simulink model "Simulacion_stepper"  (R2025b)
settings: Solver=ode4  StartTime=0.0  StopTime=Time_simulation  FixedStep=1/frecuency_simulation  RelTol=1e-3
InitFcn:
  | %%InitFcn();
StopFcn:
  | %%FinishFcn
model workspace (MAT data in the model file):
  Ts_stepper = 0.001
values from neighbouring files (symbols this model uses):
  B = motor_params.B_internal    [bode.m]    (also in current_observer.m = 0.0005; discretizacion.m = [ 1/L, 0; ekf_4_estados.m = params.B; obs_ctrl_back_emf_ext.m = [1/L 0)
  frecuency_simulation = 10e3    (= 10000)    [InitFcn.m]
  J = motor_params.J_internal    [bode.m]    (also in current_observer.m = 0.008; ekf_4_estados.m = params.J; obs_ctrl_back_emf_ext.m = 0.008; obs_y_contrl_back_emd.m = 0.008)
  Ke = 0.0055    [current_observer.m]    (also in ekf_4_estados.m = params.Ke; observer.m = Pvec(3); salient_motor.m = 0.0066)
  Ki_d = PI_dq_params.Ki_d_salient    [bode.m]
  Ki_q = PI_dq_params.Ki_q_salient    [bode.m]
  Ki_w = (wn_w^2)*J_var/Kt    [Barrido_B.m]    (also in Barrido_J.m; bode.m = PI_MTPA_params.Ki_w)
  Kp_d = PI_dq_params.Kp_d_salient    [bode.m]
  Kp_q = PI_dq_params.Kp_q_salient    [bode.m]
  Kp_w = (2*shi_w*wn_w*J_var)/Kt    [Barrido_B.m]    (also in Barrido_J.m; bode.m = PI_MTPA_params.Kp_w)
  Kt = Nr*Ke    (= 0.275)    [current_observer.m]    (also in ekf_4_estados.m = params.Kt; frecuencia_max.m = 0.33; observer.m = Pvec(4); salient_motor.m = 0.33)
  L = place(A', C', 10*eig(A)).'    [current_observer.m]    (also in desfase.m = lags(k); discretizacion.m = 0.01; frecuencia_max.m = 0.006; obs_ctrl_back_emf_ext.m = 0.006)
  P = motor_params.P    [bode.m]    (also in ekf_4_estados.m = P_pred; frecuencia_max.m = 50; salient_motor.m = 50)
  R = motor_params.R    [bode.m]    (also in current_observer.m = 3.4; discretizacion.m = 3.4; ekf_4_estados.m = params.R; frecuencia_max.m = 3.4)
  sample_time = 1/frecuency_simulation    (= 0.0001)    [InitFcn.m]
  Ts_current = 1/f_current    (= 0.0001)    [InitFcn.m]
  Ts_Wm = Ts_current*10    (= 0.001)    [InitFcn.m]
  Vdc = 24    [InitFcn.m]    (also in frecuencia_max.m = 12)
undefined symbols (not defined in the file or in its folder): DiscIntNeverNeededParam, EKF_params, motor_params, RI_base
libraries: simulink x8, mcbeeMathTransformLib x3, spspowerguiLib x1
(part 1 of 5)
settings Model: DataTypeOverride=Off  SimulationMode=accelerator  Creator=PC  LastModifiedBy=damia
settings DataIOCC: Decimation=20
settings OptimizationCC: OptimizeBlockIOStorage=off  SimCompilerOptimization=on  OptimizeDataStoreBuffers=off  BusAssignmentInplaceUpdate=off  UseRowMajorAlgorithm=on
settings DebuggingCC: SFUnexpectedBacktrackingDiag=warning  SFNoUnconditionalDefaultTransitionDiag=warning  UnderSpecifiedDimensionMsg=warning
settings RTWCC: GenerateReport=on  BuildConfiguration=Debug  LaunchReport=on
settings CodeAppCC: ForceParamTrailComments=on  MATLABSourceComments=on  EnableCustomComments=on
settings GRTTargetCC: MultiInstanceErrorCode=Warning  CombineSignalStateStructs=on  SupportVariableSizeSignals=on
settings SimscapeCC: ExplicitSolverDiagnosticOptions=none

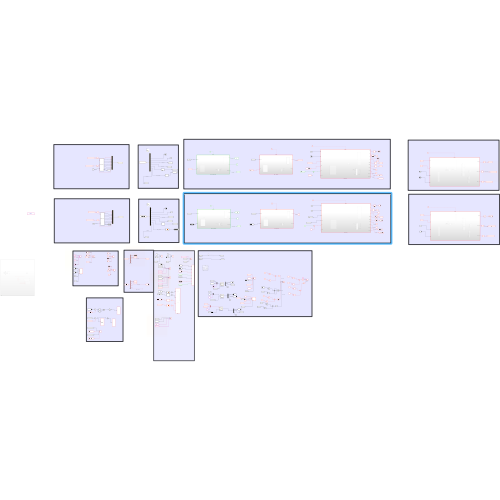
[thumbnail: Simulink's stored preview of the top-level diagram]
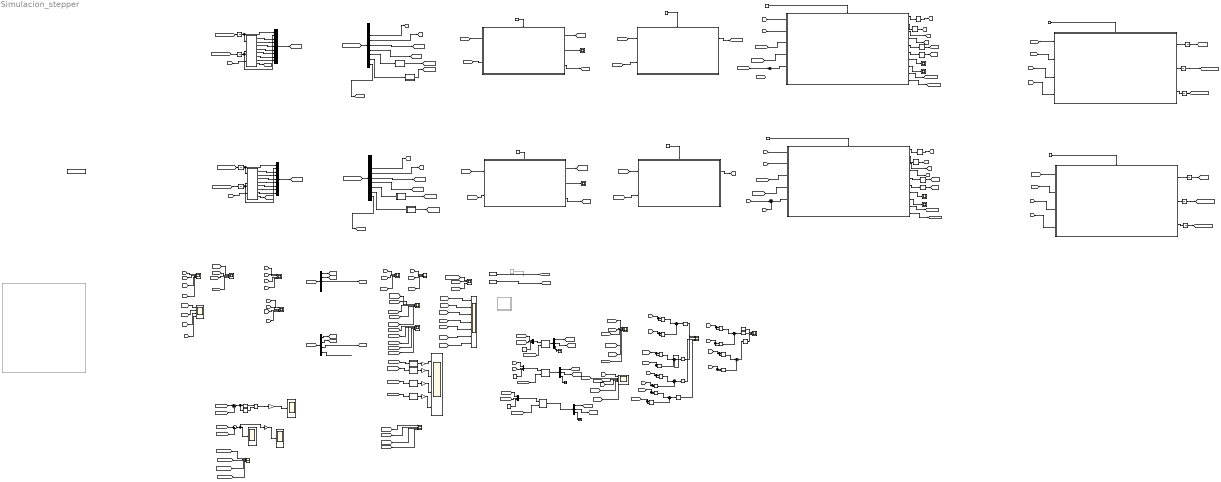
== system Simulacion_stepper ==
  note: Vab
      | Iab,
      | Te(N*m),
      | We(rad/s),
      | Theta_e(rad)
  note: Vab
      | Iab,
      | Te(N*m),
      | We(rad/s),
      | Theta_e(rad)
  Atan1 : Trigonometry  Operator=atan2
  Clarke to Park Angle Transform : mcbeeMathTransformLib/Clarke to Park Angle Transform  AxisAlignment=D-axis  UseWithEmbedded=off  PhaseInput=Two inputs  ThetaInput=Sine and Cosine electrical position  AngleInput=Per-unit  N_points=1024
      settings: LibrarySourceBlock=|
      | ee_sl_lib/Mathematical
      | Transforms/Clarke to Park
      | Angle Transform
  Clarke to Park Angle Transform1 : mcbeeMathTransformLib/Clarke to Park Angle Transform  AxisAlignment=D-axis  UseWithEmbedded=off  PhaseInput=Two inputs  ThetaInput=Sine and Cosine electrical position  AngleInput=Per-unit  N_points=1024
      settings: LibrarySourceBlock=|
      | ee_sl_lib/Mathematical
      | Transforms/Clarke to Park
      | Angle Transform
  Constant1 : Constant  Value=Vdc
  Constant11 : Constant  Value=0  OutDataTypeStr=double
  Constant2 : Constant  Value=0  OutDataTypeStr=double
  Constant6 : Constant  Value=0  OutDataTypeStr=double
  Cos1 : Trigonometry  Operator=cos
  Demux : Demux  Outputs=9
  Demux1 : Demux  Outputs=3
  Demux2 : Demux  Outputs=3
  Demux3 : Demux  Outputs=9
  Demux5 : Demux  Outputs=3
  Function-Call Generator : FunctionCallGenerator  SampleTime=EKF_params.Ts
  Function-Call Generator1 : FunctionCallGenerator  SampleTime=EKF_params.Ts
  Function-Call Generator10 : FunctionCallGenerator  Commented=on  SampleTime=1/1000
  Function-Call Generator13 : FunctionCallGenerator  SampleTime=RI_base.Ts
  Function-Call Generator2 : FunctionCallGenerator  SampleTime=RI_base.Ts
  Function-Call Generator3 : FunctionCallGenerator  SampleTime=Ts_current
  Function-Call Generator4 : FunctionCallGenerator  SampleTime=Ts_current
  Function-Call Generator5 : FunctionCallGenerator  SampleTime=Ts_Wm
  Function-Call Generator6 : FunctionCallGenerator  SampleTime=Ts_Wm
  Gain{1,25..26,28,30} (5 alike) : Gain  Gain=180/pi
  Gain2 : Gain  Gain=motor_params.P
  Iab : Scope  NumInputPorts=4
      settings: ActiveDisplayYMinimum=-2.7580893331915077  ActiveDisplayYMaximum=5.9277803516478356  DataLoggingVariableName=ScopeData8
  Id : Scope  NumInputPorts=6
      settings: ActiveDisplayYMinimum=-0.42609115554446897  ActiveDisplayYMaximum=0.9985187345386608  DataLoggingVariableName=ScopeData2
  Idq : Scope  NumInputPorts=4
      settings: ActiveDisplayYMinimum=-1  ActiveDisplayYMaximum=1  DataLoggingVariableName=ScopeData6
  Imag : Scope  NumInputPorts=4
      settings: ActiveDisplayYMinimum=-0.27016077029893221  ActiveDisplayYMaximum=2.4314469326903905  DataLoggingVariableName=ScopeData2
  Iq : Scope  NumInputPorts=6
      settings: ActiveDisplayYMinimum=-0.66469283994282913  ActiveDisplayYMaximum=2.8527838782953632  DataLoggingVariableName=Iq
  Level-2 MATLAB S-Function : M-S-Function  FunctionName=PMSM_salient  Parameters=motor_params
  Level-2 MATLAB S-Function1 : M-S-Function  FunctionName=PMSM_salient  Parameters=motor_params
  MATLAB Function1 : MATLAB Function  TreatAsAtomicUnit=on
  MATLAB Function10 : MATLAB Function  TreatAsAtomicUnit=on
  MATLAB Function12 : MATLAB Function  TreatAsAtomicUnit=on
  MATLAB Function14 : MATLAB Function  TreatAsAtomicUnit=on
  MATLAB Function3 : MATLAB Function  TreatAsAtomicUnit=on
  MATLAB Function4 : MATLAB Function  TreatAsAtomicUnit=on
  MATLAB Function5 : MATLAB Function  TreatAsAtomicUnit=on
  MATLAB Function9 : MATLAB Function  TreatAsAtomicUnit=on
  Motor 1  Speed PR : Subsystem  TreatAsAtomicUnit=on
  Motor 2  Speed PR : Subsystem  TreatAsAtomicUnit=on
  Motor 2 PI Speed MTPA : Subsystem  TreatAsAtomicUnit=on
  Motor 2 PI Speed MTPA2 : Subsystem  TreatAsAtomicUnit=on
  Motor 2 PI dq : Subsystem  TreatAsAtomicUnit=on
  Motor 2 PI dq1 : Subsystem  TreatAsAtomicUnit=on
  Mux1 : Mux  Inputs=9
  Mux2 : Mux  Inputs=3
  Mux3 : Mux  Inputs=3
  Mux4 : Mux  Inputs=9
  Mux5 : Mux  Inputs=3
  Park to Clarke Angle Transform : mcbeeMathTransformLib/Park to Clarke Angle Transform  AxisAlignment=D-axis  UseWithEmbedded=off  PhaseInput=Two inputs  ThetaInput=Sine and Cosine electrical position  AngleInput=Per-unit  N_points=1024
      settings: LibrarySourceBlock=|
      | ee_sl_lib/Mathematical
      | Transforms/Park to Clarke
      | Angle Transform
  Product{,1..7,14..17} (12 alike) : Product
  Rate Transition{1..8} (8 alike) : RateTransition
  Scope{1,3,7..8,10..11,14..15,18} (9 alike) : Scope
      Scope1 settings: ActiveDisplayYMinimum=-1  ActiveDisplayYMaximum=1  DataLoggingVariableName=ScopeData13
      Scope10 settings: ActiveDisplayYMinimum=-28.272805787309412  ActiveDisplayYMaximum=20.9806919386897  DataLoggingVariableName=ScopeData15
      Scope11 settings: ActiveDisplayYMinimum=-12246.521454579266  ActiveDisplayYMaximum=6009.4483803605362  DataLoggingVariableName=ScopeData18
      Scope14 settings: ActiveDisplayYMinimum=-21.63251363440429  ActiveDisplayYMaximum=12.126898976697245
      Scope15 settings: ActiveDisplayYMinimum=-3.7842974391773385  ActiveDisplayYMaximum=5.2532390639650686
      Scope18 settings: ActiveDisplayYMinimum=-1  ActiveDisplayYMaximum=1  DataLoggingVariableName=ScopeData14
      Scope3 settings: ActiveDisplayYMinimum=-25.99232285218147  ActiveDisplayYMaximum=26.712868682551036  DataLoggingVariableName=ScopeData10
      Scope7 settings: ActiveDisplayYMinimum=-28.272805787309412  ActiveDisplayYMaximum=20.9806919386897  DataLoggingVariableName=ScopeData11
      Scope8 settings: ActiveDisplayYMinimum=-25.99232285218147  ActiveDisplayYMaximum=26.712868682551036  DataLoggingVariableName=ScopeData17
  Scope12 : Scope  NumInputPorts=3
      settings: ActiveDisplayYMinimum=-0.46724306234141394  ActiveDisplayYMaximum=0.44219800668257625  DataLoggingVariableName=ScopeData2
  Scope2 : Scope  NumInputPorts=7
      settings: ActiveDisplayYMinimum=-3.4057486074692189  ActiveDisplayYMaximum=17.21642789399754
  Scope4 : Scope  NumInputPorts=4
      settings: ActiveDisplayYMinimum=-0.031489749327242751  ActiveDisplayYMaximum=0.031489751273901176  DataLoggingVariableName=ScopeData12
  Scope5 : Scope  NumInputPorts=5
      settings: ActiveDisplayYMinimum=-0.11835861027046617  ActiveDisplayYMaximum=0.88581558269388327
  Scope6 : Scope  NumInputPorts=3
      settings: ActiveDisplayYMinimum=-2.72699  ActiveDisplayYMaximum=4.80249
  Scope9 : Scope  NumInputPorts=4
      settings: ActiveDisplayYMinimum=-0.078542596521209512  ActiveDisplayYMaximum=0.051240487920084017  DataLoggingVariableName=ScopeData16
  Sin1 : Trigonometry
  Sqrt{,1..5} (6 alike) : Sqrt
  Subsystem1 : Subsystem  Commented=on
  Sum{1..6,13..14} (8 alike) : Sum  Inputs=|++
  Sum7 : Sum  Inputs=|+-
  Sum9 : Sum  Inputs=|+-
  Te : Scope  NumInputPorts=5
      settings: ActiveDisplayYMinimum=-0.031497005621000287  ActiveDisplayYMaximum=0.029140494372188255  DataLoggingVariableName=ScopeData2
  Terminator1 : Terminator
  Terminator2 : Terminator
  Terminator3 : Terminator
  Theta_e : Scope  NumInputPorts=4
      settings: ActiveDisplayYMinimum=-308.70038006354309  ActiveDisplayYMaximum=202.06256848293435
  Triggered Subsystem : Subsystem  Commented=on  TreatAsAtomicUnit=on
  Triggered Subsystem1 : Subsystem  TreatAsAtomicUnit=on  DataTypeOverride=Single
  Triggered Subsystem2 : Subsystem  TreatAsAtomicUnit=on  DataTypeOverride=Single
  Unit Delay{1..10} (10 alike) : UnitDelay  SampleTime=-1  HasFrameUpgradeWarning=on
  Vab : Scope  NumInputPorts=4
      settings: ActiveDisplayYMinimum=-4.125  ActiveDisplayYMaximum=4.125  DataLoggingVariableName=ScopeData7
  Valpha_betha : Scope  NumInputPorts=4
      settings: ActiveDisplayYMinimum=-2.9999999999999991  ActiveDisplayYMaximum=27  DataLoggingVariableName=ScopeData3
  Vdq : Scope  NumInputPorts=4
      settings: ActiveDisplayYMinimum=-12.409092353940933  ActiveDisplayYMaximum=27.623166475378763  DataLoggingVariableName=ScopeData5
  Vmag : Scope  NumInputPorts=3
      settings: ActiveDisplayYMinimum=-2.9178979771997589  ActiveDisplayYMaximum=26.435321997466648  DataLoggingVariableName=ScopeData3
  We : Scope  NumInputPorts=3
      settings: ActiveDisplayYMinimum=72.111947362295382  ActiveDisplayYMaximum=388.0476080584769  DataLoggingVariableName=ScopeData4
  Wm_ref : FromWorkspace  VariableName=Wm_ref  Interpolate=off  OutputAfterFinalValue=Holding final value
  Wm_ref3 : FromWorkspace  VariableName=Tl  Interpolate=off  OutputAfterFinalValue=Holding final value
  ekf_4var1 : Demux
  ekf_4var2 : Demux  Outputs=5
  powergui : spspowerguiLib/powergui  Priority=1  SimulationMode=Discrete  SampleTime=1/frecuency_simulation  frequency=60  Iterations=50  frequencyindice=0  Pbase=100e6  ErrMax=1e-4  UnitsV=kV  UnitsW=MW  buscounter=0  FunctionMessages=off  echomessages=off  EnableUseOfTLC=off  CurrentSourceSwitches=off  DisableSnubberDevices=off  DisableRonSwitches=off  DisableVfSwitches=off  DisplayEquations=off  AutomaticDiscreteSolvers=off  SolverType=Tustin/Backward Euler (TBE)  Interpol=off  ExternalGateDelay=off  methode=off  Ts=100  x0status=blocks  SPID=on  SwTol=0  HookPort=off  NonlinearTolerance=1e-4  nMaxIteration=100  ContinueOnMaxIteration=off  RestoreLinks=warning  ResistiveCurrentMeasurement=off  Frange=[0:2:500]  Ylog=off  Xlog=on  ShowGrid=off  save=off  variable=ZData  structure=0  ZoomFFT=off  StartTime=0.0  cycles=1  DisplayStyle=1  fundamental=60  FreqAxis=off  MaxFrequency=1000  frequencyindicesteady=1  RmsSteady=1  display=off
  tag scope: T_ref=global, T_ref_M1=global, Te_planta_M1=global, Te_planta_M2=global, We_planta_M1=global, We_planta_M2=global, Wm_planta_M1=global, Wm_planta_M2=global, theta_e_planta_M1=global, theta_e_planta_M2=global
  wires:
  [Te_planta_M1] -> Te/1
  [We_planta_M1] -> We/2
  [Vd_M1] -> Vdq/1  "Vd_M1"
  [Iq_M1] -> Idq/2  "Iq_M1"
  [Id_M1] -> Idq/1  "Id_M1"
  [Vq_M1] -> Vdq/2  "Vq_M1"
  [Ia_M1] -> Mux2/1
  [Ib_M1] -> Mux2/2
  Constant11/1 -> Mux2/3
  Mux2/1 -> Clarke to Park Angle Transform1/1
  Clarke to Park Angle Transform1/1 -> Demux2/1
  Demux2/3 -> Terminator1/1
  [Iq_M1] -> Iq/1
  [Iq_ref_M1] -> Iq/2
  [Iq_M1] -> Product/2, Product/1
  [Id_M1] -> Product1/2, Product1/1
  Product/1 -> Sum13/1
  Product1/1 -> Sum13/2
  Sum13/1 -> Sqrt/1
  Sqrt/1 -> Imag/1  "I_sat_obs_M1"
  Product3/1 -> Sum14/2
  Sum14/1 -> Sqrt1/1
  [Vq_M1] -> Product2/2, Product2/1
  [Vd_M1] -> Product3/2, Product3/1
  Sqrt1/1 -> Vmag/2  "V_sat_M1"
  Product2/1 -> Sum14/1
  Function-Call Generator/1 -> Triggered Subsystem1/Trigger
  [Te_planta_M2] -> Te/2
  [theta_m_planta_M1] -> Scope5/1
  [theta_m_ref] -> Scope5/3
  [Ia_M2] -> Scope6/2
  [Ia_M1] -> Scope6/1
  [Ib_M1] -> Scope12/1
  [Ib_M2] -> Scope12/2
  [Valpha_M1] -> Valpha_betha/1  "Valpha_M1"
  [Vbetha_M1] -> Valpha_betha/2  "Vbetha_M1"
  Constant1/1 -> Vmag/1
  [Vb_M1] -> Vab/2  "Vb_M1"
  [Va_M1] -> Vab/1  "Va_M1"
  [Valpha_M2] -> Valpha_betha/3  "Valpha_M2"
  [Vbetha_M2] -> Valpha_betha/4  "Vbetha_M2"
  [Ib_M1] -> Iab/2  "Ib_M1"
  [Ia_M1] -> Iab/1  "Ia_M1"
  [Vd_M2] -> Vdq/3  "Vd_M2"
  [Vq_M2] -> Vdq/4  "Vq_M2"
  [Id_M2] -> Idq/3  "Id_M2"
  [Iq_M2] -> Idq/4  "Iq_M2"
  [Iq_M2] -> Iq/4
  [Iq_ref_M2] -> Iq/5
  Product4/1 -> Sum1/1
  [Id_M2] -> Product5/2, Product5/1
  Sum1/1 -> Sqrt2/1
  [Iq_M2] -> Product4/2, Product4/1
  Product5/1 -> Sum1/2
  Product7/1 -> Sum2/2
  [Vq_M2] -> Product6/2, Product6/1
  Sum2/1 -> Sqrt3/1
  [Vd_M2] -> Product7/2, Product7/1
  Product6/1 -> Sum2/1
  Sqrt3/1 -> Vmag/3  "V_sat_M2"
  MATLAB Function3/1(y) -> [theta_m_planta_M2]
  MATLAB Function4/1(y) -> [theta_e_planta_M2]
  [Wm_ref] -> Scope2/1
  Function-Call Generator4/1 -> Motor 2 PI dq/Trigger
  Function-Call Generator5/1 -> Motor 2 PI Speed MTPA/Trigger
  [Wm_ref] -> Motor 2 PI Speed MTPA/1(Wm_ref)
  Motor 2 PI dq/3(Id) -> [Id_M2]
  Motor 2 PI dq/4(Iq) -> [Iq_M2]
  [We_planta_M2] -> We/3
  [var_stepper_M2] -> Demux/1
  Demux/3 -> [Ia_M2]
  Demux/4 -> [Ib_M2]
  [We_planta_M0] -> We/1
  [Va_M2] -> Vab/4  "Va_M2"
  [Vb_M2] -> Vab/3  "Vb_M2"
  [Ia_M2] -> Iab/3  "Ia_M2"
  [Ib_M2] -> Iab/4  "Ib_M2"
  ekf_4var1/2 -> [Iq_obs_M2]  "Iq_obs_M2"
  [x_ekf_5var_M2] -> ekf_4var1/1
  ekf_4var1/3 -> [Wm_obs_M2]  "Wm_obs_M2"
  ekf_4var1/1 -> [Id_obs_M2]  "Id_obs_M2"
  [Ia_obs_M2] -> Scope6/3
  [Ib_obs_M2] -> Scope12/3
  [Id_M1] -> Id/1
  [Id_M2] -> Id/4
  [Ib_M2] -> Mux5/2
  Mux5/1 -> Clarke to Park Angle Transform/1
  [Ia_M2] -> Mux5/1
  Constant6/1 -> Mux5/3
  Clarke to Park Angle Transform/1 -> Demux1/1
  Demux1/3 -> Terminator2/1
  Demux2/1 -> [Id_real_M1]  "Id_real_M1"
  Demux2/2 -> [Iq_real_M1]  "Iq_real_M1"
  Demux1/1 -> [Id_real_M2]  "Id_real_M2"
  Demux1/2 -> [Iq_real_M2]  "Iq_real_M2"
  [Iq_real_M1] -> Iq/3
  [Iq_real_M2] -> Iq/6
  [Id_real_M2] -> Id/6
  Product15/1 -> Sum5/2
  [Id_real_M1] -> Product15/2, Product15/1
  [Iq_real_M1] -> Product14/2, Product14/1
  Sum5/1 -> Sqrt4/1
  Product14/1 -> Sum5/1
  Sum6/1 -> Sqrt5/1
  [Id_real_M2] -> Product17/2, Product17/1
  [Iq_real_M2] -> Product16/2, Product16/1
  Product17/1 -> Sum6/2
  Product16/1 -> Sum6/1
  Sqrt4/1 -> Imag/2  "I_sat_real_M1"
  Sqrt5/1 -> Imag/4  "I_sat_real_M2"
  Sqrt2/1 -> Imag/3  "I_sat_obs_M2"
  [theta_e_obs_M2] -> MATLAB Function14/1(u)
  [theta_e_obs_M1] -> MATLAB Function12/1(u)
  [theta_e_planta_M2] -> MATLAB Function10/1(u)
  [theta_e_planta_M1] -> MATLAB Function9/1(u)
  MATLAB Function10/1(y) -> Gain26/1
  MATLAB Function14/1(y) -> Gain30/1
  MATLAB Function12/1(y) -> Gain28/1
  MATLAB Function9/1(y) -> Gain25/1
  Gain25/1 -> Theta_e/1
  Gain26/1 -> Theta_e/2
  Gain28/1 -> Theta_e/3
  Gain30/1 -> Theta_e/4
  [theta_e_planta_M2] -> Clarke to Park Angle Transform/2
  [theta_e_planta_M1] -> Clarke to Park Angle Transform1/2
  [Wm_obs_M1] -> Sum7/2
  [Wm_planta_M1] -> Sum7/1
  Sum7/1 -> Gain2/1, Scope15/1
  Level-2 MATLAB S-Function/1 -> Mux4/3
  Level-2 MATLAB S-Function/2 -> Mux4/4
  Mux4/1 -> [var_stepper_M2]
  Level-2 MATLAB S-Function/3 -> Mux4/5
  Level-2 MATLAB S-Function/4 -> Mux4/6
  Level-2 MATLAB S-Function/5 -> Mux4/7
  Level-2 MATLAB S-Function/6 -> Mux4/8
  Level-2 MATLAB S-Function/7 -> Mux4/9
  Demux/5 -> [Wm_planta_M2]  "Wm_real_M2"
  Demux/6 -> [We_planta_M2]
  Demux/7 -> MATLAB Function3/1(u)
  Demux/8 -> MATLAB Function4/1(u)  "theta_e_planta_M2"
  Demux/9 -> [Te_planta_M2]  "Te_planta_M2"
  [Wm_planta_M1] -> Scope2/2
  [Wm_planta_M2] -> Scope2/5
  [Wm_obs_M2] -> Scope2/6
  [Wm_filt_M2] -> Scope2/7
  [Id_obs_M2] -> Mux3/1
  Mux3/1 -> Park to Clarke Angle Transform/1
  Constant2/1 -> Mux3/3
  [Iq_obs_M2] -> Mux3/2
  [theta_e_planta_M2] -> Park to Clarke Angle Transform/2
  Demux5/2 -> [Ib_obs_M2]  "Ib_obs_M2"
  Demux5/1 -> [Ia_obs_M2]  "Ia_obs_M2"
  Demux5/3 -> Terminator3/1
  Park to Clarke Angle Transform/1 -> Demux5/1
  [Vbetha_M2] -> Unit Delay5/1
  Unit Delay5/1 -> Level-2 MATLAB S-Function/2, Mux4/2
  [Valpha_M2] -> Unit Delay10/1
  Unit Delay10/1 -> Mux4/1, Level-2 MATLAB S-Function/1
  [Tx_hat_M1] -> Te/3
  [Ia_M2] -> Motor 2 PI dq/1(Ia)
  [Ib_M2] -> Motor 2 PI dq/2(Ib)
  Function-Call Generator10/1 -> ?
  Wm_ref/1 -> [Wm_ref]
  Motor 2 PI dq/7(Vd_hfi) -> Scope3/1  "Vd_HFI_M2"
  Motor 2 PI dq/8(Vq_hfi) -> Scope7/1  "Vq_HFI_M2"
  [Wm_planta_M2] -> Motor 2 PI Speed MTPA/2(Wm)
  [theta_m_planta_M2] -> Scope5/4
  Motor 2 PI Speed MTPA/2(T_pi) -> Scope18/1
  Motor 2 PI Speed MTPA/1(T_ref) -> [T_ref]  "T_ref_M2"
  Level-2 MATLAB S-Function/8 -> [Tdtm_M2]  "Tdtm_M2"
  [Tdtm_M2] -> Te/5
  [Tl] -> Level-2 MATLAB S-Function/3  "Tl_M2"
  [Tx_hat_M2] -> Scope9/3
  [Tdtm_M2] -> Scope9/1
  [Tl] -> Scope9/2
  [Tx_obs_M2] -> Scope9/4
  [Id_real_M1] -> Id/3
  [Id_ref_M2] -> Id/5
  Wm_ref3/1 -> [Tl]
  Triggered Subsystem1/1(kf_5var2) -> Unit Delay1/1
  Unit Delay1/1 -> [x_ekf_5var_M2]
  Motor 2 PI dq/5(Valpha) -> Rate Transition5/1
  Rate Transition5/1 -> [Valpha_M2]
  Motor 2 PI dq/6(Vbetha) -> Rate Transition6/1
  Rate Transition6/1 -> [Vbetha_M2]
  Rate Transition7/1 -> [Vd_M2]  "Vd_M2"
  Motor 2 PI dq/1(Vd) -> Rate Transition7/1
  Motor 2 PI dq/2(Vq) -> Rate Transition8/1
  Rate Transition8/1 -> [Vq_M2]  "Vq_M2"
  [Valpha_M2] -> Triggered Subsystem1/1(Va)
  Gain2/1 -> Scope11/1
  [Vbetha_M2] -> Triggered Subsystem1/2(Vb)
  [Ia_M2] -> Triggered Subsystem1/3(Ia)
  [Ib_M2] -> Triggered Subsystem1/4(Ib)
  [Wm_planta_M2] -> Motor 2 PI dq/3(Wm)
  Motor 2 PI Speed MTPA/3(Wm_filt_out) -> [Wm_filt_M2]  "Wm_filt_M2"
  Motor 2 PI dq/9(Id_ref_out) -> [Id_ref_M2]  "Id_ref_M2"
  Motor 2 PI dq/10(Iq_ref_out) -> [Iq_ref_M2]  "Iq_ref_M2"
  [theta_e_planta_M2] -> Motor 2 PI dq/4(Theta)
  Triggered Subsystem1/3(theta_e_hat) -> Unit Delay2/1
  Unit Delay2/1 -> [theta_e_obs_M2]
  Triggered Subsystem1/2(theta_m_hat) -> Unit Delay6/1
  Unit Delay6/1 -> [theta_m_obs_M2]  "theta_m_obs_M2"
  [theta_m_obs_M2] -> Scope5/5
  [theta_ref] -> Scope5/2
  Motor 2  Speed PR/1(T_res) -> [T_res_M2]  "T_res_M2"
  [Wm_ref] -> Motor 2  Speed PR/1(Wm_ref)
  [Wm_planta_M2] -> Motor 2  Speed PR/2(Wm)
  Function-Call Generator13/1 -> Motor 2  Speed PR/Trigger
  [Tdtm_M2] -> Scope4/3
  [T_res_M2] -> Scope4/4
  [T_ref] -> Sum4/1
  Sum4/1 -> Motor 2 PI dq/5(T_ref)
  Rate Transition3/1 -> [Vd_M1]  "Vd_M1"
  [Wm_obs_M1] -> Motor 2 PI Speed MTPA2/2(Wm)
  Motor 2 PI Speed MTPA2/3(Wm_filt_out) -> [Wm_filt_M1]  "Wm_filt_M1"
  Mux1/1 -> [var_stepper_M1]
  [Ib_M1] -> Motor 2 PI dq1/2(Ib)
  [Ib_M1] -> Triggered Subsystem2/4(Ib)
  Motor 2 PI dq1/2(Vq) -> Rate Transition4/1
  Demux3/5 -> [Wm_planta_M1]  "Wm_real_M1"
  Level-2 MATLAB S-Function1/1 -> Mux1/3
  [Vbetha_M1] -> Triggered Subsystem2/2(Vb)
  Motor 2 PI dq1/5(Valpha) -> Rate Transition1/1
  Triggered Subsystem2/2(theta_m_hat) -> Unit Delay9/1
  [theta_e_obs_M1] -> Motor 2 PI dq1/4(Theta)
  MATLAB Function1/1(y) -> [theta_m_planta_M1]
  Motor 2 PI dq1/10(Iq_ref_out) -> [Iq_ref_M1]  "Iq_ref_M1"
  MATLAB Function5/1(y) -> [theta_e_planta_M1]
  Function-Call Generator6/1 -> Motor 2 PI Speed MTPA2/Trigger
  Unit Delay8/1 -> Level-2 MATLAB S-Function1/2, Mux1/2
  Level-2 MATLAB S-Function1/3 -> Mux1/5
  Triggered Subsystem2/1(kf_5var2) -> Unit Delay3/1
  Level-2 MATLAB S-Function1/8 -> [Tdtm_M1]  "Tdtm_M1"
  Unit Delay9/1 -> [theta_m_obs_M1]  "theta_m_obs_M1"
  Demux3/7 -> MATLAB Function1/1(u)
  Level-2 MATLAB S-Function1/2 -> Mux1/4
  Motor 2 PI dq1/6(Vbetha) -> Rate Transition2/1
  [Valpha_M1] -> Triggered Subsystem2/1(Va)
  Function-Call Generator3/1 -> Motor 2 PI dq1/Trigger
  Rate Transition2/1 -> [Vbetha_M1]
  Level-2 MATLAB S-Function1/5 -> Mux1/7
  [Vbetha_M1] -> Unit Delay8/1
  Function-Call Generator1/1 -> Triggered Subsystem2/Trigger
  Motor 2 PI Speed MTPA2/2(T_pi) -> Scope1/1
  Demux3/8 -> MATLAB Function5/1(u)  "theta_e_planta_M1"
  Rate Transition4/1 -> [Vq_M1]  "Vq_M1"
  Unit Delay3/1 -> [x_ekf_5var_M1]
  Motor 1  Speed PR/1(T_res) -> [T_res_M1]  "T_res_M1"
  Motor 2 PI Speed MTPA2/1(T_ref) -> [T_ref_M1]  "T_ref_M1"
  [Wm_ref] -> Motor 1  Speed PR/1(Wm_ref)
  Demux3/9 -> [Te_planta_M1]  "Te_planta_M1"
  [Wm_obs_M1] -> Motor 1  Speed PR/2(Wm)
  Demux3/3 -> [Ia_M1]
  Motor 2 PI dq1/7(Vd_hfi) -> Scope8/1  "Vd_HFI_M1"
  [Wm_obs_M1] -> Motor 2 PI dq1/3(Wm)
  [Tl] -> Level-2 MATLAB S-Function1/3  "Tl_M1"
  Motor 2 PI dq1/4(Iq) -> [Iq_M1]
  [Ia_M1] -> Triggered Subsystem2/3(Ia)
  Unit Delay4/1 -> Mux1/1, Level-2 MATLAB S-Function1/1
  Demux3/4 -> [Ib_M1]
  Motor 2 PI dq1/8(Vq_hfi) -> Scope10/1  "Vq_HFI_M1"
  Unit Delay7/1 -> [theta_e_obs_M1]
  Level-2 MATLAB S-Function1/6 -> Mux1/8
  [Wm_ref] -> Motor 2 PI Speed MTPA2/1(Wm_ref)  "Wm_ref"
  Triggered Subsystem2/3(theta_e_hat) -> Unit Delay7/1
  [Ia_M1] -> Motor 2 PI dq1/1(Ia)
  [T_ref_M1] -> Sum3/1
  Level-2 MATLAB S-Function1/4 -> Mux1/6
  Motor 2 PI dq1/1(Vd) -> Rate Transition3/1
  [var_stepper_M1] -> Demux3/1
  Sum3/1 -> Motor 2 PI dq1/5(T_ref)
  Demux3/6 -> [We_planta_M1]  "We_real_M1"
  [Valpha_M1] -> Unit Delay4/1
  Function-Call Generator2/1 -> Motor 1  Speed PR/Trigger
  Rate Transition1/1 -> [Valpha_M1]
  Level-2 MATLAB S-Function1/7 -> Mux1/9
  Motor 2 PI dq1/3(Id) -> [Id_M1]
  Motor 2 PI dq1/9(Id_ref_out) -> [Id_ref_M1]  "Id_ref_M1"
  [Id_ref_M1] -> Id/2
  [x_ekf_5var_M1] -> ekf_4var2/1
  ekf_4var2/3 -> [Wm_obs_M1]  "Wm_obs_M1"
  ekf_4var2/1 -> [Id_obs_M1]  "Id_obs_M1"
  ekf_4var2/2 -> [Iq_obs_M1]  "Iq_obs_M1"
  [Tx_hat_M2] -> Te/4
  [Wm_filt_M1] -> Scope2/4
  [Wm_obs_M1] -> Scope2/3
  Sum9/1 -> Cos1/1, Sin1/1
  Sin1/1 -> Atan1/1
  Cos1/1 -> Atan1/2
  Atan1/1 -> Gain1/1
  [theta_e_obs_M1] -> Sum9/2
  Gain1/1 -> Scope14/1
  [theta_e_planta_M1] -> Sum9/1
  [Tdtm_M1] -> Scope4/1
  [T_res_M1] -> Scope4/2
  ekf_4var1/4 -> ?  "theta_e_obs_M2"
  [T_res_M2] -> Sum4/2

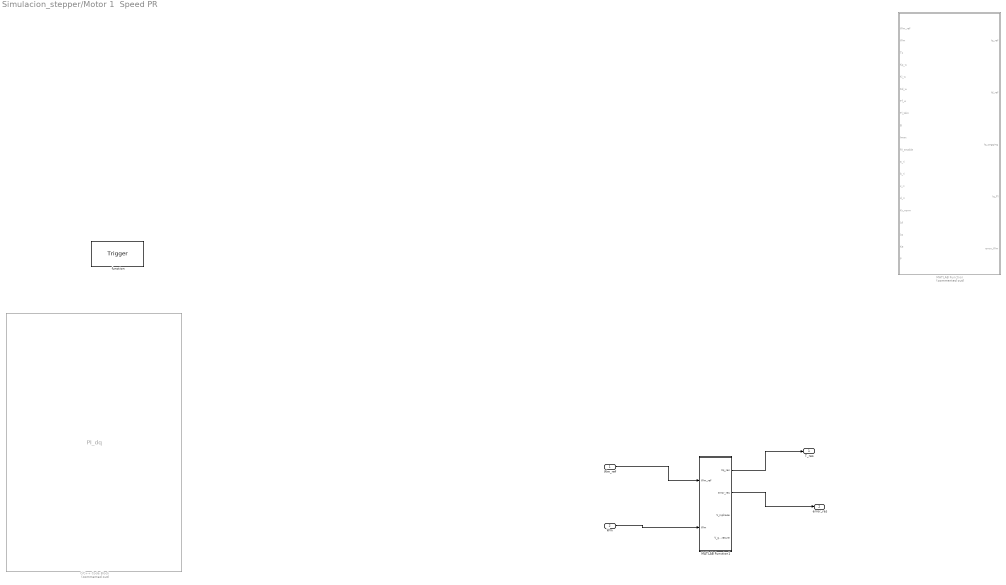
== system Simulacion_stepper/Motor 1  Speed PR ==
  Wm_ref : Inport
  Wm : Inport  Port=2
  function : TriggerPort  TriggerType=function-call  VariantControl=(inherit)  SampleTime=1/100
  C/C++ Code Block : S-Function  Commented=on  FunctionName=PI_dq  SFunctionModules=PI_dq_wrapper.c  SFunctionDeploymentMode=off  EnableBusSupport=off  mask(S-Function Builder){}
      mask help: Simulink:masks:SFunctionBuilder_MD
      mask init:
      | val = [[.9  0.75 0.75 1 1 .9 .9 1]',[1 1 0.75 0.75 .9 .9 1 .9]'];try , sys = get_param(gcb,'SfunBuilderFcnName');if isempty(sys), sys = get_param(gcb,'FunctionName'); end,catch, sys = get_param(gcb,'FunctionName'); end
      settings: CopyFcn=set_param(gcbh,'LinkStatus','none')  OpenFcn=sfunctionwizard(gcbh)
      mask Display:
      | plot(val(:,1),val(:,2))
      | disp(sys)
      | port_label('input',1,sprintf('%s', 'Ia'),'interpreter','tex')
      | port_label('input',2,sprintf('%s', 'Ib'),'interpreter','tex')
      | port_label('input',3,sprintf('%s', 'Wm\_ref'),'interpreter','tex')
      | port_label('input',4,sprintf('%s', 'Wm\_ext'),'interpreter','tex')
      | port_label('input',5,sprintf('%s', 'Kp\_current'),'interpreter','tex')
      | port_label('input',6,sprintf('%s', 'Ki\_current'),'interpreter','tex')
      | port_label('input',7,sprintf('%s', 'Kd\_current'),'interpreter','tex')
      | port_label('input',8,sprintf('%s', 'sample\_time\_ext'),'interpreter','tex')
      | port_label('input',9,sprintf('%s', 'Vdc\_ext'),'interpreter','tex')
      | port_label('input',10,sprintf('%s', 'R\_ext'),'interpreter','tex')
      | port_label('input',11,sprintf('%s', 'Ld\_ext'),'interpreter','tex')
      | port_label('input',12,sprintf('%s', 'Lq\_ext'),'interpreter','tex')
      | port_label('input',13,sprintf('%s', 'Ke\_ext'),'interpreter','tex')
      | port_label('input',14,sprintf('%s', 'Theta\_ext'),'interpreter','tex')
      | port_label('input',15,sprintf('%s', 'Kp\_wm'),'interpreter','tex')
      | port_label('input',16,sprintf('%s', 'Ki\_wm'),'interpreter','tex')
      | port_label('input',17,sprintf('%s', 'Tl\_Tdm'),'interpreter','tex')
      | port_label('input',18,sprintf('%s', 'B'),'interpreter','tex')
      | port_label('input',19,sprintf('%s', 'Kt\_ext'),'interpreter','tex')
      | port_label('output',1,sprintf('%s', 'Ud'),'interpreter','tex')
      | port_label('output',2,sprintf('%s', 'Uq'),'interpreter','tex')
      | port_label('output',3,sprintf('%s', 'Id'),'interpreter','tex')
      | port_label('output',4,sprintf('%s', 'Iq'),'interpreter','tex')
      | port_label('output',5,sprintf('%s', 'Iq\_ref\_aux'),'interpreter','tex')
  MATLAB Function : MATLAB Function  Commented=on  TreatAsAtomicUnit=on
  MATLAB Function1 : MATLAB Function  TreatAsAtomicUnit=on
  T_res : Outport
  error_res : Outport  Port=2
  wires:
  MATLAB Function1/1(Vq_res) -> T_res/1
  Wm_ref/1 -> MATLAB Function1/1(Wm_ref)
  Wm/1 -> MATLAB Function1/2(Wm)
  MATLAB Function1/2(error_res) -> error_res/1

== system Simulacion_stepper/Motor 2  Speed PR ==
  Wm_ref : Inport
  Wm : Inport  Port=2
  function : TriggerPort  TriggerType=function-call  VariantControl=(inherit)  SampleTime=1/100
  C/C++ Code Block : S-Function  Commented=on  FunctionName=PI_dq  SFunctionModules=PI_dq_wrapper.c  SFunctionDeploymentMode=off  EnableBusSupport=off  mask(S-Function Builder){}
      mask help: Simulink:masks:SFunctionBuilder_MD
      mask init: same as Simulacion_stepper/Motor 1  Speed PR/C/C++ Code Block
      settings: CopyFcn=set_param(gcbh,'LinkStatus','none')  OpenFcn=sfunctionwizard(gcbh)
      mask Display:
      | plot(val(:,1),val(:,2))
      | disp(sys)
      | port_label('input',1,sprintf('%s', 'Ia'),'interpreter','tex')
      | port_label('input',2,sprintf('%s', 'Ib'),'interpreter','tex')
      | port_label('input',3,sprintf('%s', 'Wm\_ref'),'interpreter','tex')
      | port_label('input',4,sprintf('%s', 'Wm\_ext'),'interpreter','tex')
      | port_label('input',5,sprintf('%s', 'Kp\_current'),'interpreter','tex')
      | port_label('input',6,sprintf('%s', 'Ki\_current'),'interpreter','tex')
      | port_label('input',7,sprintf('%s', 'Kd\_current'),'interpreter','tex')
      | port_label('input',8,sprintf('%s', 'sample\_time\_ext'),'interpreter','tex')
      | port_label('input',9,sprintf('%s', 'Vdc\_ext'),'interpreter','tex')
      | port_label('input',10,sprintf('%s', 'R\_ext'),'interpreter','tex')
      | port_label('input',11,sprintf('%s', 'Ld\_ext'),'interpreter','tex')
      | port_label('input',12,sprintf('%s', 'Lq\_ext'),'interpreter','tex')
      | port_label('input',13,sprintf('%s', 'Ke\_ext'),'interpreter','tex')
      | port_label('input',14,sprintf('%s', 'Theta\_ext'),'interpreter','tex')
      | port_label('input',15,sprintf('%s', 'Kp\_wm'),'interpreter','tex')
      | port_label('input',16,sprintf('%s', 'Ki\_wm'),'interpreter','tex')
      | port_label('input',17,sprintf('%s', 'Tl\_Tdm'),'interpreter','tex')
      | port_label('input',18,sprintf('%s', 'B'),'interpreter','tex')
      | port_label('input',19,sprintf('%s', 'Kt\_ext'),'interpreter','tex')
      | port_label('output',1,sprintf('%s', 'Ud'),'interpreter','tex')
      | port_label('output',2,sprintf('%s', 'Uq'),'interpreter','tex')
      | port_label('output',3,sprintf('%s', 'Id'),'interpreter','tex')
      | port_label('output',4,sprintf('%s', 'Iq'),'interpreter','tex')
      | port_label('output',5,sprintf('%s', 'Iq\_ref\_aux'),'interpreter','tex')
  MATLAB Function : MATLAB Function  Commented=on  TreatAsAtomicUnit=on
  MATLAB Function1 : MATLAB Function  TreatAsAtomicUnit=on
  T_res : Outport
  error_res : Outport  Port=2
  wires:
  MATLAB Function1/1(Vq_res) -> T_res/1
  Wm_ref/1 -> MATLAB Function1/1(Wm_ref)
  Wm/1 -> MATLAB Function1/2(Wm)
  MATLAB Function1/2(error_res) -> error_res/1

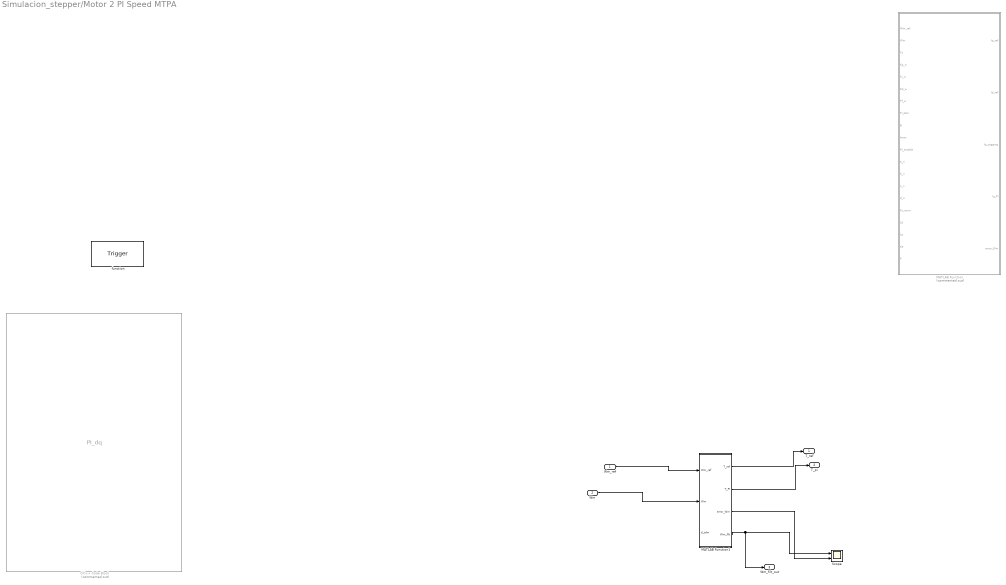
== system Simulacion_stepper/Motor 2 PI Speed MTPA ==
  Wm_ref : Inport
  Wm : Inport  Port=2
  function : TriggerPort  TriggerType=function-call  VariantControl=(inherit)  SampleTime=1/100
  C/C++ Code Block : S-Function  Commented=on  FunctionName=PI_dq  SFunctionModules=PI_dq_wrapper.c  SFunctionDeploymentMode=off  EnableBusSupport=off  mask(S-Function Builder){}
      mask help: Simulink:masks:SFunctionBuilder_MD
      mask init: same as Simulacion_stepper/Motor 1  Speed PR/C/C++ Code Block
      settings: CopyFcn=set_param(gcbh,'LinkStatus','none')  OpenFcn=sfunctionwizard(gcbh)
      mask Display:
      | plot(val(:,1),val(:,2))
      | disp(sys)
      | port_label('input',1,sprintf('%s', 'Ia'),'interpreter','tex')
      | port_label('input',2,sprintf('%s', 'Ib'),'interpreter','tex')
      | port_label('input',3,sprintf('%s', 'Wm\_ref'),'interpreter','tex')
      | port_label('input',4,sprintf('%s', 'Wm\_ext'),'interpreter','tex')
      | port_label('input',5,sprintf('%s', 'Kp\_current'),'interpreter','tex')
      | port_label('input',6,sprintf('%s', 'Ki\_current'),'interpreter','tex')
      | port_label('input',7,sprintf('%s', 'Kd\_current'),'interpreter','tex')
      | port_label('input',8,sprintf('%s', 'sample\_time\_ext'),'interpreter','tex')
      | port_label('input',9,sprintf('%s', 'Vdc\_ext'),'interpreter','tex')
      | port_label('input',10,sprintf('%s', 'R\_ext'),'interpreter','tex')
      | port_label('input',11,sprintf('%s', 'Ld\_ext'),'interpreter','tex')
      | port_label('input',12,sprintf('%s', 'Lq\_ext'),'interpreter','tex')
      | port_label('input',13,sprintf('%s', 'Ke\_ext'),'interpreter','tex')
      | port_label('input',14,sprintf('%s', 'Theta\_ext'),'interpreter','tex')
      | port_label('input',15,sprintf('%s', 'Kp\_wm'),'interpreter','tex')
      | port_label('input',16,sprintf('%s', 'Ki\_wm'),'interpreter','tex')
      | port_label('input',17,sprintf('%s', 'Tl\_Tdm'),'interpreter','tex')
      | port_label('input',18,sprintf('%s', 'B'),'interpreter','tex')
      | port_label('input',19,sprintf('%s', 'Kt\_ext'),'interpreter','tex')
      | port_label('output',1,sprintf('%s', 'Ud'),'interpreter','tex')
      | port_label('output',2,sprintf('%s', 'Uq'),'interpreter','tex')
      | port_label('output',3,sprintf('%s', 'Id'),'interpreter','tex')
      | port_label('output',4,sprintf('%s', 'Iq'),'interpreter','tex')
      | port_label('output',5,sprintf('%s', 'Iq\_ref\_aux'),'interpreter','tex')
  MATLAB Function : MATLAB Function  Commented=on  TreatAsAtomicUnit=on
  MATLAB Function1 : MATLAB Function  TreatAsAtomicUnit=on
  Scope : Scope  NumInputPorts=2
      settings: ActiveDisplayYMinimum=-0.005920462093646885  ActiveDisplayYMaximum=0.021595753043081149  DataLoggingVariableName=ScopeData9
  T_ref : Outport
  T_pi : Outport  Port=2
  Wm_filt_out : Outport  Port=3
  wires:
  MATLAB Function1/1(T_ref) -> T_ref/1
  Wm_ref/1 -> MATLAB Function1/1(Wm_ref)
  Wm/1 -> MATLAB Function1/2(Wm)
  MATLAB Function1/3(error_Wm) -> Scope/2
  MATLAB Function1/2(T_PI) -> T_pi/1
  MATLAB Function1/4(Wm_filt) -> Wm_filt_out/1, Scope/1

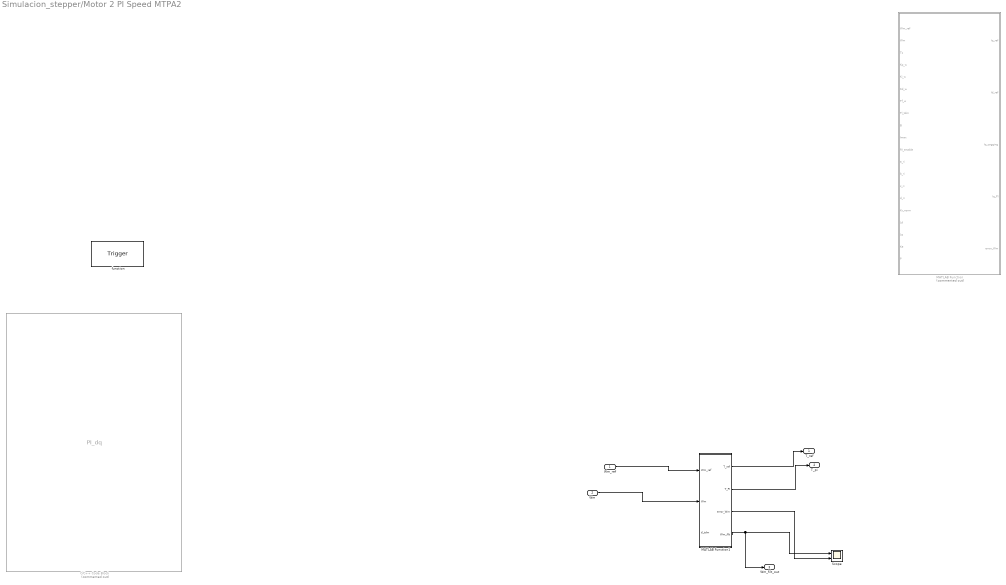
== system Simulacion_stepper/Motor 2 PI Speed MTPA2 ==
  Wm_ref : Inport
  Wm : Inport  Port=2
  function : TriggerPort  TriggerType=function-call  VariantControl=(inherit)  SampleTime=1/100
  C/C++ Code Block : S-Function  Commented=on  FunctionName=PI_dq  SFunctionModules=PI_dq_wrapper.c  SFunctionDeploymentMode=off  EnableBusSupport=off  mask(S-Function Builder){}
      mask help: Simulink:masks:SFunctionBuilder_MD
      mask init: same as Simulacion_stepper/Motor 1  Speed PR/C/C++ Code Block
      settings: CopyFcn=set_param(gcbh,'LinkStatus','none')  OpenFcn=sfunctionwizard(gcbh)
      mask Display:
      | plot(val(:,1),val(:,2))
      | disp(sys)
      | port_label('input',1,sprintf('%s', 'Ia'),'interpreter','tex')
      | port_label('input',2,sprintf('%s', 'Ib'),'interpreter','tex')
      | port_label('input',3,sprintf('%s', 'Wm\_ref'),'interpreter','tex')
      | port_label('input',4,sprintf('%s', 'Wm\_ext'),'interpreter','tex')
      | port_label('input',5,sprintf('%s', 'Kp\_current'),'interpreter','tex')
      | port_label('input',6,sprintf('%s', 'Ki\_current'),'interpreter','tex')
      | port_label('input',7,sprintf('%s', 'Kd\_current'),'interpreter','tex')
      | port_label('input',8,sprintf('%s', 'sample\_time\_ext'),'interpreter','tex')
      | port_label('input',9,sprintf('%s', 'Vdc\_ext'),'interpreter','tex')
      | port_label('input',10,sprintf('%s', 'R\_ext'),'interpreter','tex')
      | port_label('input',11,sprintf('%s', 'Ld\_ext'),'interpreter','tex')
      | port_label('input',12,sprintf('%s', 'Lq\_ext'),'interpreter','tex')
      | port_label('input',13,sprintf('%s', 'Ke\_ext'),'interpreter','tex')
      | port_label('input',14,sprintf('%s', 'Theta\_ext'),'interpreter','tex')
      | port_label('input',15,sprintf('%s', 'Kp\_wm'),'interpreter','tex')
      | port_label('input',16,sprintf('%s', 'Ki\_wm'),'interpreter','tex')
      | port_label('input',17,sprintf('%s', 'Tl\_Tdm'),'interpreter','tex')
      | port_label('input',18,sprintf('%s', 'B'),'interpreter','tex')
      | port_label('input',19,sprintf('%s', 'Kt\_ext'),'interpreter','tex')
      | port_label('output',1,sprintf('%s', 'Ud'),'interpreter','tex')
      | port_label('output',2,sprintf('%s', 'Uq'),'interpreter','tex')
      | port_label('output',3,sprintf('%s', 'Id'),'interpreter','tex')
      | port_label('output',4,sprintf('%s', 'Iq'),'interpreter','tex')
      | port_label('output',5,sprintf('%s', 'Iq\_ref\_aux'),'interpreter','tex')
  MATLAB Function : MATLAB Function  Commented=on  TreatAsAtomicUnit=on
  MATLAB Function1 : MATLAB Function  TreatAsAtomicUnit=on
  Scope : Scope  NumInputPorts=2
      settings: ActiveDisplayYMinimum=-0.005920462093646885  ActiveDisplayYMaximum=0.021595753043081149  DataLoggingVariableName=ScopeData9
  T_ref : Outport
  T_pi : Outport  Port=2
  Wm_filt_out : Outport  Port=3
  wires:
  MATLAB Function1/1(T_ref) -> T_ref/1
  Wm_ref/1 -> MATLAB Function1/1(Wm_ref)
  Wm/1 -> MATLAB Function1/2(Wm)
  MATLAB Function1/3(error_Wm) -> Scope/2
  MATLAB Function1/2(T_PI) -> T_pi/1
  MATLAB Function1/4(Wm_filt) -> Wm_filt_out/1, Scope/1

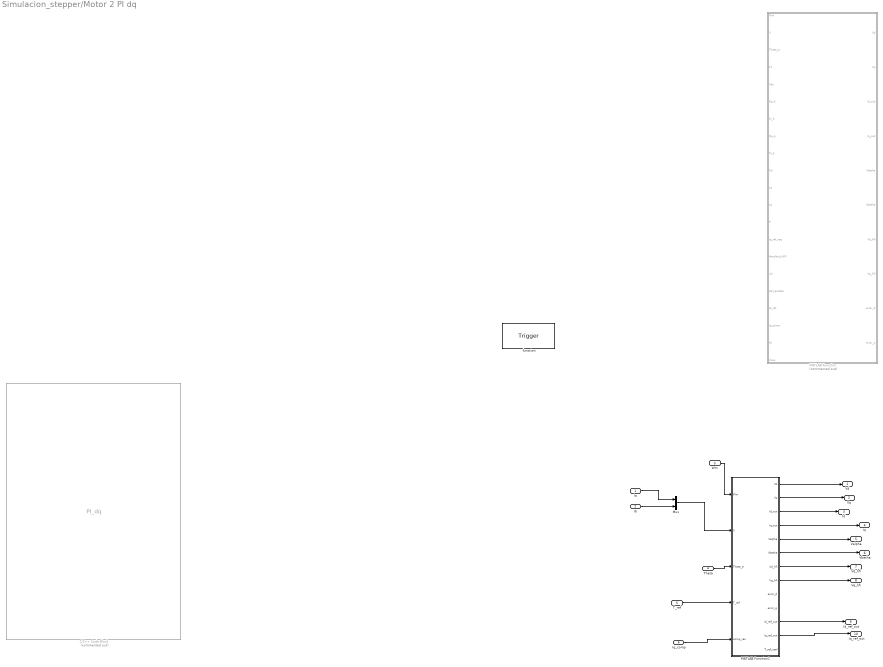
== system Simulacion_stepper/Motor 2 PI dq ==
  Ia : Inport  PortDimensions=1
  Ib : Inport  Port=2  PortDimensions=1
  Wm : Inport  Port=3
  Theta : Inport  Port=4
  T_ref : Inport  Port=5
  Iq_comp : Inport  Port=6
  function : TriggerPort  TriggerType=function-call  VariantControl=(inherit)  SampleTime=1/100
  C/C++ Code Block : S-Function  Commented=on  FunctionName=PI_dq  SFunctionModules=PI_dq_wrapper.c  SFunctionDeploymentMode=off  EnableBusSupport=off  mask(S-Function Builder){}
      mask help: Simulink:masks:SFunctionBuilder_MD
      mask init: same as Simulacion_stepper/Motor 1  Speed PR/C/C++ Code Block
      settings: CopyFcn=set_param(gcbh,'LinkStatus','none')  OpenFcn=sfunctionwizard(gcbh)
      mask Display:
      | plot(val(:,1),val(:,2))
      | disp(sys)
      | port_label('input',1,sprintf('%s', 'Ia'),'interpreter','tex')
      | port_label('input',2,sprintf('%s', 'Ib'),'interpreter','tex')
      | port_label('input',3,sprintf('%s', 'Wm\_ref'),'interpreter','tex')
      | port_label('input',4,sprintf('%s', 'Wm\_ext'),'interpreter','tex')
      | port_label('input',5,sprintf('%s', 'Kp\_current'),'interpreter','tex')
      | port_label('input',6,sprintf('%s', 'Ki\_current'),'interpreter','tex')
      | port_label('input',7,sprintf('%s', 'Kd\_current'),'interpreter','tex')
      | port_label('input',8,sprintf('%s', 'sample\_time\_ext'),'interpreter','tex')
      | port_label('input',9,sprintf('%s', 'Vdc\_ext'),'interpreter','tex')
      | port_label('input',10,sprintf('%s', 'R\_ext'),'interpreter','tex')
      | port_label('input',11,sprintf('%s', 'Ld\_ext'),'interpreter','tex')
      | port_label('input',12,sprintf('%s', 'Lq\_ext'),'interpreter','tex')
      | port_label('input',13,sprintf('%s', 'Ke\_ext'),'interpreter','tex')
      | port_label('input',14,sprintf('%s', 'Theta\_ext'),'interpreter','tex')
      | port_label('input',15,sprintf('%s', 'Kp\_wm'),'interpreter','tex')
      | port_label('input',16,sprintf('%s', 'Ki\_wm'),'interpreter','tex')
      | port_label('input',17,sprintf('%s', 'Tl\_Tdm'),'interpreter','tex')
      | port_label('input',18,sprintf('%s', 'B'),'interpreter','tex')
      | port_label('input',19,sprintf('%s', 'Kt\_ext'),'interpreter','tex')
      | port_label('output',1,sprintf('%s', 'Ud'),'interpreter','tex')
      | port_label('output',2,sprintf('%s', 'Uq'),'interpreter','tex')
      | port_label('output',3,sprintf('%s', 'Id'),'interpreter','tex')
      | port_label('output',4,sprintf('%s', 'Iq'),'interpreter','tex')
      | port_label('output',5,sprintf('%s', 'Iq\_ref\_aux'),'interpreter','tex')
  MATLAB Function : MATLAB Function  Commented=on  TreatAsAtomicUnit=on
  MATLAB Function1 : MATLAB Function  TreatAsAtomicUnit=on
  Mux : Mux  Inputs=2
  Vd : Outport  PortDimensions=1
  Vq : Outport  Port=2  PortDimensions=1
  Id : Outport  Port=3
  Iq : Outport  Port=4
  Valpha : Outport  Port=5
  Vbetha : Outport  Port=6
  Vd_hfi : Outport  Port=7
  Vq_hfi : Outport  Port=8
  Id_ref_out : Outport  Port=9
  Iq_ref_out : Outport  Port=10
  wires:
  MATLAB Function1/1(Vd) -> Vd/1
  Wm/1 -> MATLAB Function1/1(Wm)
  Ia/1 -> Mux/1
  Ib/1 -> Mux/2
  Mux/1 -> MATLAB Function1/2(X)
  Theta/1 -> MATLAB Function1/3(Theta_e)
  MATLAB Function1/2(Vq) -> Vq/1
  MATLAB Function1/3(Id_out) -> Id/1
  MATLAB Function1/4(Iq_out) -> Iq/1
  MATLAB Function1/5(Valpha) -> Valpha/1
  MATLAB Function1/6(Vbetha) -> Vbetha/1
  MATLAB Function1/7(Vd_hfi) -> Vd_hfi/1
  MATLAB Function1/8(Vq_hfi) -> Vq_hfi/1
  T_ref/1 -> MATLAB Function1/4(T_ref)
  MATLAB Function1/11(Id_ref_out) -> Id_ref_out/1
  MATLAB Function1/12(Iq_ref_out) -> Iq_ref_out/1
  Iq_comp/1 -> MATLAB Function1/5(comp_res)

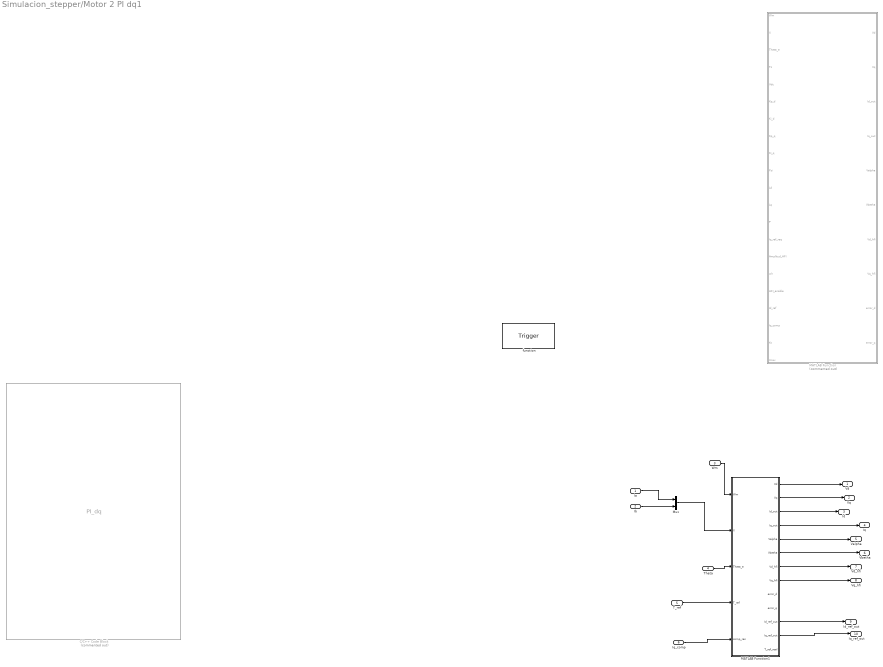
== system Simulacion_stepper/Motor 2 PI dq1 ==
  Ia : Inport  PortDimensions=1
  Ib : Inport  Port=2  PortDimensions=1
  Wm : Inport  Port=3
  Theta : Inport  Port=4
  T_ref : Inport  Port=5
  Iq_comp : Inport  Port=6
  function : TriggerPort  TriggerType=function-call  VariantControl=(inherit)  SampleTime=1/100
  C/C++ Code Block : S-Function  Commented=on  FunctionName=PI_dq  SFunctionModules=PI_dq_wrapper.c  SFunctionDeploymentMode=off  EnableBusSupport=off  mask(S-Function Builder){}
      mask help: Simulink:masks:SFunctionBuilder_MD
      mask init: same as Simulacion_stepper/Motor 1  Speed PR/C/C++ Code Block
      settings: CopyFcn=set_param(gcbh,'LinkStatus','none')  OpenFcn=sfunctionwizard(gcbh)
      mask Display:
      | plot(val(:,1),val(:,2))
      | disp(sys)
      | port_label('input',1,sprintf('%s', 'Ia'),'interpreter','tex')
      | port_label('input',2,sprintf('%s', 'Ib'),'interpreter','tex')
      | port_label('input',3,sprintf('%s', 'Wm\_ref'),'interpreter','tex')
      | port_label('input',4,sprintf('%s', 'Wm\_ext'),'interpreter','tex')
      | port_label('input',5,sprintf('%s', 'Kp\_current'),'interpreter','tex')
      | port_label('input',6,sprintf('%s', 'Ki\_current'),'interpreter','tex')
      | port_label('input',7,sprintf('%s', 'Kd\_current'),'interpreter','tex')
      | port_label('input',8,sprintf('%s', 'sample\_time\_ext'),'interpreter','tex')
      | port_label('input',9,sprintf('%s', 'Vdc\_ext'),'interpreter','tex')
      | port_label('input',10,sprintf('%s', 'R\_ext'),'interpreter','tex')
      | port_label('input',11,sprintf('%s', 'Ld\_ext'),'interpreter','tex')
      | port_label('input',12,sprintf('%s', 'Lq\_ext'),'interpreter','tex')
      | port_label('input',13,sprintf('%s', 'Ke\_ext'),'interpreter','tex')
      | port_label('input',14,sprintf('%s', 'Theta\_ext'),'interpreter','tex')
      | port_label('input',15,sprintf('%s', 'Kp\_wm'),'interpreter','tex')
      | port_label('input',16,sprintf('%s', 'Ki\_wm'),'interpreter','tex')
      | port_label('input',17,sprintf('%s', 'Tl\_Tdm'),'interpreter','tex')
      | port_label('input',18,sprintf('%s', 'B'),'interpreter','tex')
      | port_label('input',19,sprintf('%s', 'Kt\_ext'),'interpreter','tex')
      | port_label('output',1,sprintf('%s', 'Ud'),'interpreter','tex')
      | port_label('output',2,sprintf('%s', 'Uq'),'interpreter','tex')
      | port_label('output',3,sprintf('%s', 'Id'),'interpreter','tex')
      | port_label('output',4,sprintf('%s', 'Iq'),'interpreter','tex')
      | port_label('output',5,sprintf('%s', 'Iq\_ref\_aux'),'interpreter','tex')
  MATLAB Function : MATLAB Function  Commented=on  TreatAsAtomicUnit=on
  MATLAB Function1 : MATLAB Function  TreatAsAtomicUnit=on
  Mux : Mux  Inputs=2
  Vd : Outport  PortDimensions=1
  Vq : Outport  Port=2  PortDimensions=1
  Id : Outport  Port=3
  Iq : Outport  Port=4
  Valpha : Outport  Port=5
  Vbetha : Outport  Port=6
  Vd_hfi : Outport  Port=7
  Vq_hfi : Outport  Port=8
  Id_ref_out : Outport  Port=9
  Iq_ref_out : Outport  Port=10
  wires:
  MATLAB Function1/1(Vd) -> Vd/1
  Wm/1 -> MATLAB Function1/1(Wm)
  Ia/1 -> Mux/1
  Ib/1 -> Mux/2
  Mux/1 -> MATLAB Function1/2(X)
  Theta/1 -> MATLAB Function1/3(Theta_e)
  MATLAB Function1/2(Vq) -> Vq/1
  MATLAB Function1/3(Id_out) -> Id/1
  MATLAB Function1/4(Iq_out) -> Iq/1
  MATLAB Function1/5(Valpha) -> Valpha/1
  MATLAB Function1/6(Vbetha) -> Vbetha/1
  MATLAB Function1/7(Vd_hfi) -> Vd_hfi/1
  MATLAB Function1/8(Vq_hfi) -> Vq_hfi/1
  T_ref/1 -> MATLAB Function1/4(T_ref)
  MATLAB Function1/11(Id_ref_out) -> Id_ref_out/1
  MATLAB Function1/12(Iq_ref_out) -> Iq_ref_out/1
  Iq_comp/1 -> MATLAB Function1/5(comp_res)

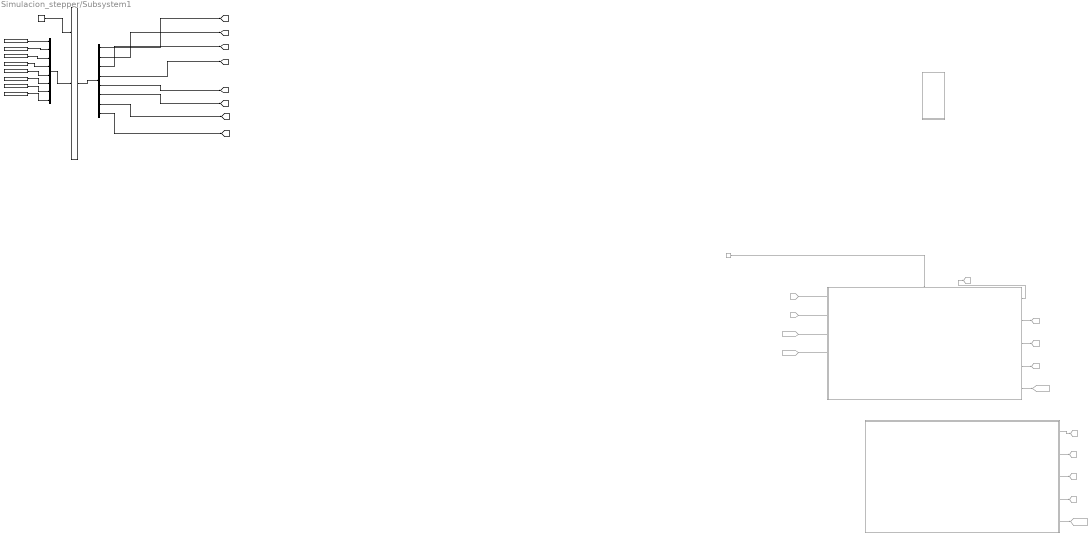
== system Simulacion_stepper/Subsystem1 ==
  note: A
  note: A
  note: A
  Constant1 : Constant
  Demux6 : Demux  Outputs=8
  From103 : From  Commented=on  GotoTag=Ib_M1
  From110 : From  Commented=on  GotoTag=Wm_ref  TagVisibility=global
  From112 : From  Commented=on  GotoTag=Wm_planta_M1  TagVisibility=global
  From98 : From  Commented=on  GotoTag=Ia_M1
  Function-Call Generator3 : FunctionCallGenerator  Commented=on  SampleTime=sample_time
  Goto14 : Goto  Commented=on  GotoTag=Vd_M2  TagVisibility=global
  Goto15 : Goto  Commented=on  GotoTag=Vq_M2  TagVisibility=global
  Goto16 : Goto  Commented=on  GotoTag=Iq_M2  TagVisibility=global
  Goto17 : Goto  Commented=on  GotoTag=Iq_ref_M2  TagVisibility=global
  Goto4 : Goto  Commented=on  GotoTag=Id_M2  TagVisibility=global
  Goto55 : Goto  Commented=on  GotoTag=Id_M1  TagVisibility=global
  Goto64 : Goto  Commented=on  GotoTag=Vd_M1  TagVisibility=global
  Goto65 : Goto  Commented=on  GotoTag=Vq_M1  TagVisibility=global
  Goto66 : Goto  Commented=on  GotoTag=Iq_M1  TagVisibility=global
  Goto68 : Goto  Commented=on  GotoTag=Iq_ref_M1  TagVisibility=global
  Multiport Switch : MultiPortSwitch  Inputs=2  SaturateOnIntegerOverflow=off  InputSameDT=off
  Mux1 : Mux  Inputs=8
  Repeating Sequence Stair : simulink/Sources/Repeating Sequence Stair  OutValues=[1 0 0 0]  tsamp=Ts_stepper  OutMin=[]  OutMax=[]  OutDataTypeStr=double  OutputDataTypeScalingMode=double  OutDataType=fixdt(0,8)  ConRadixGroup=Best Precision: Vector-wise  OutScaling=2^-12
  Repeating Sequence Stair1 : simulink/Sources/Repeating Sequence Stair  OutValues=[1 0 1 0]  tsamp=Ts_stepper  OutMin=[]  OutMax=[]  OutDataTypeStr=double  OutputDataTypeScalingMode=double  OutDataType=fixdt(0,8)  ConRadixGroup=Best Precision: Vector-wise  OutScaling=2^-12
  Repeating Sequence Stair10 : simulink/Sources/Repeating Sequence Stair  OutValues=[0 0 0 1]  tsamp=Ts_stepper  OutMin=[]  OutMax=[]  OutDataTypeStr=double  OutputDataTypeScalingMode=double  OutDataType=fixdt(0,8)  ConRadixGroup=Best Precision: Vector-wise  OutScaling=2^-12
  Repeating Sequence Stair11 : simulink/Sources/Repeating Sequence Stair  OutValues=[1 0 0 1]  tsamp=Ts_stepper  OutMin=[]  OutMax=[]  OutDataTypeStr=double  OutputDataTypeScalingMode=double  OutDataType=fixdt(0,8)  ConRadixGroup=Best Precision: Vector-wise  OutScaling=2^-12
  Repeating Sequence Stair2 : simulink/Sources/Repeating Sequence Stair  OutValues=[0 0 1 0]  tsamp=Ts_stepper  OutMin=[]  OutMax=[]  OutDataTypeStr=double  OutputDataTypeScalingMode=double  OutDataType=fixdt(0,8)  ConRadixGroup=Best Precision: Vector-wise  OutScaling=2^-12
  Repeating Sequence Stair3 : simulink/Sources/Repeating Sequence Stair  OutValues=[0 1 1 0]  tsamp=Ts_stepper  OutMin=[]  OutMax=[]  OutDataTypeStr=double  OutputDataTypeScalingMode=double  OutDataType=fixdt(0,8)  ConRadixGroup=Best Precision: Vector-wise  OutScaling=2^-12
  Repeating Sequence Stair8 : simulink/Sources/Repeating Sequence Stair  OutValues=[0 1 0 0]  tsamp=Ts_stepper  OutMin=[]  OutMax=[]  OutDataTypeStr=double  OutputDataTypeScalingMode=double  OutDataType=fixdt(0,8)  ConRadixGroup=Best Precision: Vector-wise  OutScaling=2^-12
  Repeating Sequence Stair9 : simulink/Sources/Repeating Sequence Stair  OutValues=[0 1 0 1]  tsamp=Ts_stepper  OutMin=[]  OutMax=[]  OutDataTypeStr=double  OutputDataTypeScalingMode=double  OutDataType=fixdt(0,8)  ConRadixGroup=Best Precision: Vector-wise  OutScaling=2^-12
  Subsystem : Subsystem  Commented=on
  Triggered Subsystem2 : Subsystem  Commented=on  TreatAsAtomicUnit=on
  Triggered Subsystem4 : Subsystem  Commented=on  TreatAsAtomicUnit=on
  wires:
  Triggered Subsystem2/4(Iq) -> Goto66/1
  Triggered Subsystem2/1(Vd) -> Goto64/1
  ? -> Triggered Subsystem4/6(Tl_Tdm)
  ? -> Triggered Subsystem2/5(Theta)
  ? -> Triggered Subsystem4/3(Wm_ref)
  Triggered Subsystem2/5(Iq_ref) -> Goto68/1
  From112/1 -> Triggered Subsystem2/4(Wm)
  Triggered Subsystem4/2(Vq) -> Goto15/1
  From98/1 -> Triggered Subsystem2/1(Ia)
  Triggered Subsystem2/2(Vq) -> Goto65/1
  ? -> Triggered Subsystem2/6(Tl_Tdm)
  From103/1 -> Triggered Subsystem2/2(Ib)
  Triggered Subsystem2/3(Id) -> Goto55/1
  From110/1 -> Triggered Subsystem2/3(Wm_ref)
  Triggered Subsystem4/3(Id) -> Goto4/1
  ? -> Triggered Subsystem4/Trigger
  Triggered Subsystem4/4(Iq) -> Goto16/1
  ? -> Triggered Subsystem4/4(Wm)
  Triggered Subsystem4/5(Iq_ref) -> Goto17/1
  ? -> Triggered Subsystem4/5(Theta)
  ? -> Triggered Subsystem4/1(Ia)
  Function-Call Generator3/1 -> Triggered Subsystem2/Trigger
  ? -> Triggered Subsystem4/2(Ib)
  Triggered Subsystem4/1(Vd) -> Goto14/1
  Demux6/2 -> [S2_M0]
  Demux6/1 -> [S1_M0]
  Repeating Sequence Stair10/1 -> Mux1/7
  Repeating Sequence Stair8/1 -> Mux1/5
  Repeating Sequence Stair9/1 -> Mux1/6
  Demux6/8 -> [S8_M0]
  Demux6/4 -> [S4_M0]
  Demux6/7 -> [S7_M0]
  Demux6/6 -> [S6_M0]
  Constant1/1 -> Multiport Switch/1
  Repeating Sequence Stair/1 -> Mux1/1
  Mux1/1 -> Multiport Switch/2
  Repeating Sequence Stair3/1 -> Mux1/4
  Repeating Sequence Stair11/1 -> Mux1/8
  Demux6/5 -> [S5_M0]
  Repeating Sequence Stair2/1 -> Mux1/3
  Repeating Sequence Stair1/1 -> Mux1/2
  Multiport Switch/1 -> Demux6/1
  Demux6/3 -> [S3_M0]

== system Simulacion_stepper/Triggered Subsystem ==
  Wm_cmd : Inport
  Trigger : TriggerPort  TriggerType=function-call  VariantControl=(inherit)
  Constant : Constant  Value=1/1000
  Constant1 : Constant  Value=0
  MATLAB Function : MATLAB Function  TreatAsAtomicUnit=on
  Wm_ref : Outport
  Alpha_ref : Outport  Port=2
  wires:
  MATLAB Function/1(Wm_ref) -> Wm_ref/1
  MATLAB Function/2(alpha_ref) -> Alpha_ref/1
  Wm_cmd/1 -> MATLAB Function/1(Wm_cmd)
  Constant/1 -> MATLAB Function/2(Ts)
  Constant1/1 -> MATLAB Function/3(slope)
